simulink model "WMMSupportingForcesGP2021b"  (R2021b)
settings: Solver=ode23t  StartTime=0.0  StopTime=inf  FixedStep=.001  RelTol=1e-3  AbsTol=1e-3
InitFcn:
  | InitializeSimulationGP
  | SimulationParametersGP
values from neighbouring files (symbols this model uses):
  B11_r_B11C = [0.23805608; 0.13201777; 0]    [InitializeSimulationGP.m]
  B11_r_B11Tc1 = [L11; 0; 0]    [InitializeSimulationGP.m]
  B11_Rot_Tc1 = eye(3)    [InitializeSimulationGP.m]
  B11cI = [0.28426000 -0.06487287 0;         -0.06487287  0.54237481 0;                   0  0          0.67891020]    [InitializeSimulationGP.m]
  B12_r_B12C = [0.60504569; 0.27199376; 0.00002484]    [InitializeSimulationGP.m]
  B12_r_B12Tc2 = [L12;0;0]    [InitializeSimulationGP.m]
  B12_Rot_Tc2 = eye(3)    [InitializeSimulationGP.m]
  B12cI = [1.18803886 -2.36786418 0.00280315;          -2.36786418 6.31493281 0.00022322;           0.00280315 0.00022322 7.40915161]    [InitializeSimulationGP.m]
  B31_r_B31C = [0.35781210 0 0]    [InitializeSimulationGP.m]
  B31_Rot_B41 = eye(3)    [InitializeSimulationGP.m]
  B31cI = diag([0.03150902 0.90735702 0.90763033])    [InitializeSimulationGP.m]
  B32_r_B32C = [0.35781210 0 0]    [InitializeSimulationGP.m]
  B32_Rot_B42 = eye(3)    [InitializeSimulationGP.m]
  B32cI = diag([0.03150902 0.90735702 0.90763033])    [InitializeSimulationGP.m]
  B41_r_B41C = [0.55785997 0 0]    [InitializeSimulationGP.m]
  B41_r_B41Tc1 = [lc1;0;0]    [InitializeSimulationGP.m]
  B41cI = diag([0.00370720 0.55759812 0.55785997])    [InitializeSimulationGP.m]
  B42_r_B42C = [0.55785997 0 0]    [InitializeSimulationGP.m]
  B42_r_B42Tc2 = [lc2; 0; 0]    [InitializeSimulationGP.m]
  B42cI = diag([0.00370720 0.55759812 0.55785997])    [InitializeSimulationGP.m]
  B52_r_B52C = [0 0 0.56802906]    [InitializeSimulationGP.m]
  B52_r_B52P32 = [lc3; 0; 0]    [InitializeSimulationGP.m]
  B52_Rot_P32 = eye(3)    [InitializeSimulationGP.m]
  B52cI = diag([0.91789884, 0.91790043, 0.00091463])    [InitializeSimulationGP.m]
  Bc1_r_Bc1B11 = [L1; 0; 0]    [InitializeSimulationGP.m]
  Bc1_r_Bc1B31 = [0;0;0]    [InitializeSimulationGP.m]
  Bc1_r_Bc1C = [0.14178771; 0.16555780; 0]    [InitializeSimulationGP.m]
  Bc1_V = [0;0;0;0;0;0]    [InitializeSimulationGP.m]
  Bc1cI = [+5.892211080 +5.476111360 -0.000019630;          +5.476111360 +28.66965601 -0.000024550;          -0.000019630 -0.000024550 +29.78955950]    [InitializeSimulationGP.m]
  Bc2_r_Bc2B12 = [L2;0;0]    [InitializeSimulationGP.m]
  Bc2_r_Bc2B32 = [0;0;0]    [InitializeSimulationGP.m]
  Bc2_r_Bc2C = [0.54319901; 0.10543875; 0]    [InitializeSimulationGP.m]
  Bc2cI = [0.48071390 0.52924041 0;          0.52924041 5.80912352 0;              0      0          5.97255351]    [InitializeSimulationGP.m]
  BC_r_BCBM = [xCA; yCA; zCA]    [SimulationParametersGP.m]
  BC_Rot_BM = eye(3)    [SimulationParametersGP.m]
  BCI = diag([100 1200 1000])    [SimulationParametersGP.m]
  beta1 = atan2d(374.261,935)*pi/180    [InitializeSimulationGP.m]
  beta2 = atan2d(45.757,373.313)*pi/180    [InitializeSimulationGP.m]
  beta3 = atan2d(139.50,1132.19)*pi/180    [InitializeSimulationGP.m]
  beta4 = atan2d(88.061,296.198)*pi/180    [InitializeSimulationGP.m]
  betaGround = 1e6    (= 1000000)    [SimulationParametersGP.m]
  BFL = 0.05    [SimulationParametersGP.m]
  BFR = 0.05    [SimulationParametersGP.m]
  BM_r_BMBMp = [0;0;0]    [SimulationParametersGP.m]
  BM_Rot_BMp = [cos(gamma) -sin(gamma) 0; sin(gamma) cos(gamma) 0; 0 0 1]    [SimulationParametersGP.m]
  BMp_r_BMpBc1 = [0.185;0;0.205]    [InitializeSimulationGP.m]
  BMp_Rot_Bc1 = [cos(alpha1) -sin(alpha1)  0;                  0            0       -1;                sin(alpha1)  cos(alpha1)  0]    [InitializeSimulationGP.m]
  BRL = 0.05    [SimulationParametersGP.m]
  BRR = 0.05    [SimulationParametersGP.m]
  cc = 0.0    (= 0)    [SimulationParametersGP.m]
  D22F = [0;0;0;0;0;0]    [InitializeSimulationGP.m]
  dT = 0.01    [SimulationParametersGP.m]
  g0 = 9.8066    [SimulationParametersGP.m]
  ground_stiffness = 1e8    (= 100000000)    [SimulationParametersGP.m]
  l1 = 1.15-cc    (= 1.15)    [SimulationParametersGP.m]
  L1 = 1.0071227324212    (= 1.00712273242)    [InitializeSimulationGP.m]
  L11 = 0.37610632101293    (= 0.376106321013)    [InitializeSimulationGP.m]
  L12 = 0.30901132665325    (= 0.309011326653)    [InitializeSimulationGP.m]
  l2 = 1.15+cc    (= 1.15)    [SimulationParametersGP.m]
  L2 = 1.132185817991    (= 1.13218581799)    [InitializeSimulationGP.m]
  lc1 = 0.745    [InitializeSimulationGP.m]
  lc2 = 0.745    [InitializeSimulationGP.m]
  mB11 = 25.52660174    [InitializeSimulationGP.m]
  mB12 = 33.92850233    [InitializeSimulationGP.m]
  mB31 = 17.36281648    [InitializeSimulationGP.m]
  mB32 = 17.36281648    [InitializeSimulationGP.m]
  mB41 = 10.34519231    [InitializeSimulationGP.m]
  mB42 = 10.34519231    [InitializeSimulationGP.m]
  mB52 = 6.73059863    [InitializeSimulationGP.m]
  mBC = 2200    [SimulationParametersGP.m]
  mBc1 = 307.29601379    [InitializeSimulationGP.m]
  mBc2 = 54.58702836    [InitializeSimulationGP.m]
  mFL = 60    [SimulationParametersGP.m]
  mFR = 60    [SimulationParametersGP.m]
  mP22 = 9.26136143    [InitializeSimulationGP.m]
  mP32 = 570.18877059    [InitializeSimulationGP.m]
  mRR = 60    [SimulationParametersGP.m]
  mw = mFL    (= 60)    [SimulationParametersGP.m]
  P22_r_P22C = [0.62192523 0 0]    [InitializeSimulationGP.m]
  P22_Rot_B52 = eye(3)    [InitializeSimulationGP.m]
  P22cI = diag([0.00662754, 1.48387017, 1.48398069])    [InitializeSimulationGP.m]
  P32_r_P32C = [0.25466704; -0.13034397; -0.01302248]    [InitializeSimulationGP.m]
  P32_r_P32D22 = [0.40499744871392; -0.13130517281345; -0.013385243295654]    [InitializeSimulationGP.m]
  P32_Rot_D22 = [1 0 0;              0 0.9707729441837 0.23999977258512;              0 -0.23999977258512 0.9707729441837]    [InitializeSimulationGP.m]
  P32cI = [46.81220713 0.38607676 -0.00453819;          0.38607676 71.92201786 -1.14320993;          -0.00453819 -1.14320993 67.38128576]    [InitializeSimulationGP.m]
  R0FL = 0.35    [SimulationParametersGP.m]
  R0FR = 0.35    [SimulationParametersGP.m]
  R0RL = 0.35    [SimulationParametersGP.m]
  R0RR = 0.35    [SimulationParametersGP.m]
  Rw = R0FL    (= 0.35)    [SimulationParametersGP.m]
  Tc1_r_Tc1Bc2 = [0.098495302558553; 0.01838181329939; 0]    [InitializeSimulationGP.m]
  Tc1_Rot_Bc2 = [cos(alpha2) -sin(alpha2) 0;                sin(alpha2)  cos(alpha2) 0;                0            0           1]    [InitializeSimulationGP.m]
  Tc2_r_Tc2P22 = [-0.048858374920227;0.36587359346146;0.035276938723102]    [InitializeSimulationGP.m]
  Tc2_Rot_P22 = [0.95853460763586 -0.27664713597974  0.0683942111482;                0.28497614981675  0.93051946315663 -0.23004808784757;                0                 0.23999977258511  0.9707729441837]    [InitializeSimulationGP.m]
  Th1A = 10*pi/180    (= 0.174532925199)    [InitializeSimulationGP.m]
  Th1B = 20*pi/180    (= 0.349065850399)    [InitializeSimulationGP.m]
  Th1f = 1    [InitializeSimulationGP.m]
  Th2A = 15*pi/180    (= 0.261799387799)    [InitializeSimulationGP.m]
  Th2B = -70*pi/180    (= -1.2217304764)    [InitializeSimulationGP.m]
  Th2f = 2    [InitializeSimulationGP.m]
  w = wFL    (= 0.875)    [SimulationParametersGP.m]
  W_r_WBc1 = [0.185;0;0.205]    [InitializeSimulationGP.m]
  W_Rot_Bc1 = [cos(alpha1) -sin(alpha1)  0;                  0            0       -1;                sin(alpha1)  cos(alpha1)  0]    [InitializeSimulationGP.m]
  x10 = 0.83    [InitializeSimulationGP.m]
  x20 = 0.83    [InitializeSimulationGP.m]
  x3A = 0.2    [InitializeSimulationGP.m]
  x3B = 0.3    [InitializeSimulationGP.m]
  x3f = 1    [InitializeSimulationGP.m]
  xCA = 0.5    [SimulationParametersGP.m]
  xf = [1;0;0;0;0;0]    [InitializeSimulationGP.m]
  yCA = 0    [SimulationParametersGP.m]
  zC = 0.45    [SimulationParametersGP.m]
  zCA = .25    (= 0.25)    [SimulationParametersGP.m]
  ztau = [0;0;0;0;0;1]    [InitializeSimulationGP.m]
undefined symbols (not defined in the file or in its folder): alphaFL_meas, alphaFR_meas, alphaRL_meas, alphaRR_meas, B11_V, B11Ftot, B12_U_Tc2, B12_V, B12Ftot, B31_r_B31B41, B31_V, B31FTot, B32_r_B32B42, B32_U_B42, B32_V, B32FTot, B41_V, B41FTot, B42_Rot_Tc2, B42_U_Tc2, B42_V, B42FTot, B52_U_P32, B52_V, B52Ftot, Bc1Tot, Bc2_Rot_B12, Bc2_Rot_B32, Bc2_U_B12, Bc2_U_B32, Bc2_V, Bc2Tot, betaC_meas, D22_V, deltaFL_cmd, deltaFL_meas, deltaFR_cmd, deltaFR_meas, deltaRL_cmd, deltaRL_meas, deltaRR_cmd, deltaRR_meas, dOmegaFL_meas, dOmegaFR_meas, dOmegaRL_meas, dOmegaRR_meas, dPsi_meas, dq1, dq11, dq12, dq2, dq21, dq22, dx1, dx2, Floor, FTot_S1, FTot_S2P, FTot_S2R, FzFL ... (+63)
libraries: sm_lib x94, nesl_utility x63, simulink x5
(part 7 of 11)

== system WMMSupportingForcesGP2021b/Mobile Manipulator in Simscape/Hydraulic manipulator, Simscape/TiltCylinderAndTiltPiston ==
  B32Aux : sm_lib/Frames and Transforms/Rigid Transform  TranslationMethod=None  TranslationStandardOffset=0  TranslationLengthUnit=m  TranslationStandardAxis=+Z  TranslationCartesianOffset=[0 0 0]  TranslationROffset=0  TranslationROffsetUnits=m  TranslationZOffset=0  TranslationZOffsetUnits=m  TranslationThetaOffset=0  TranslationThetaOffsetUnits=deg  RotationMethod=StandardAxis  RotationAngleUnits=deg  RotationStandardAxis=+Y  RotationAngle=90  RotationArbitraryAxis=[0 0 1]  FollAlignAxisA=+X  BaseAlignAxisA=+Y  FollAlignAxisB=+Y  BaseAlignAxisB=+Z  RotationSequenceAxes=FollowerAxes  RotationSequence=XYX  RotationSequenceAngles=[0 0 0]  RotationSequenceAnglesUnits=deg  RotationMatrix=[1 0 0; 0 1 0; 0 0 1]
  B42Aux : sm_lib/Frames and Transforms/Rigid Transform  TranslationMethod=None  TranslationStandardOffset=0  TranslationLengthUnit=m  TranslationStandardAxis=+Z  TranslationCartesianOffset=[0 0 0]  TranslationROffset=0  TranslationROffsetUnits=m  TranslationZOffset=0  TranslationZOffsetUnits=m  TranslationThetaOffset=0  TranslationThetaOffsetUnits=deg  RotationMethod=StandardAxis  RotationAngleUnits=deg  RotationStandardAxis=+Y  RotationAngle=-90  RotationArbitraryAxis=[0 0 1]  FollAlignAxisA=+X  BaseAlignAxisA=+Y  FollAlignAxisB=+Y  BaseAlignAxisB=+Z  RotationSequenceAxes=FollowerAxes  RotationSequence=XYX  RotationSequenceAngles=[0 0 0]  RotationSequenceAnglesUnits=deg  RotationMatrix=[1 0 0; 0 1 0; 0 0 1]
  PS-Sim2 : nesl_utility/PS-Simulink Converter  PhysicalDomain=network_engine_domain  SubClassName=ps_output  LeftPortType=input  RightPortType=output  PseudoPeriodic=off  Frequencies=[]  Unit=inherit  AffineConversion=off
      settings: SourceProductBaseCode=PW,SS
  Tilt cylinder rotation (q21) : sm_lib/Joints/Revolute Joint  JointMode=Normal  SenseConstraintForce=off  SenseConstraintForceX=off  SenseConstraintForceY=off  SenseConstraintForceZ=off  SenseConstraintTorque=off  SenseConstraintTorqueX=off  SenseConstraintTorqueY=off  SenseConstraintTorqueZ=off  SenseTotalForce=off  SenseTotalForceX=off  SenseTotalForceY=off  SenseTotalForceZ=off  SenseTotalTorque=off  SenseTotalTorqueX=off  SenseTotalTorqueY=off  SenseTotalTorqueZ=off  CompositeWrenchDir=FollowerOnBase  CompositeWrenchFrame=BaseFrame  EquilibriumPosition=0  EquilibriumPositionUnits=deg  SpringStiffness=0  SpringStiffnessUnits=N*m/deg  DampingCoefficient=0  DampingCoefficientUnits=N*m/(deg/s)  TorqueActuationMode=NoTorque  MotionActuationMode=ComputedMotion  SensePosition=off  SenseVelocity=off  SenseAcceleration=off  SenseTorqueForce=off  SenseLowerLimitTorqueForce=off  SenseUpperLimitTorqueForce=off  LowerLimitSpecify=off  LowerLimitBound=-90  LowerLimitBoundUnits=deg  LowerLimitStiffness=1e4  LowerLimitStiffnessUnits=N*m/deg  LowerLimitDamping=10  LowerLimitDampingUnits=N*m/(deg/s)  LowerLimitTransitionRegionWidth=0.1  LowerLimitTransitionRegionWidthUnits=deg  UpperLimitSpecify=off  UpperLimitBound=90  UpperLimitBoundUnits=deg  UpperLimitStiffness=1e4  UpperLimitStiffnessUnits=N*m/deg  UpperLimitDamping=10  UpperLimitDampingUnits=N*m/(deg/s)  UpperLimitTransitionRegionWidth=0.1  UpperLimitTransitionRegionWidthUnits=deg  PositionTargetSpecify=off  PositionTargetPriority=High  PositionTargetValue=0  PositionTargetValueUnits=deg  VelocityTargetSpecify=off  VelocityTargetPriority=High  VelocityTargetValue=0  VelocityTargetValueUnits=deg/s
  Tilt piston rotation (q22) : sm_lib/Joints/Revolute Joint  JointMode=Normal  SenseConstraintForce=off  SenseConstraintForceX=off  SenseConstraintForceY=off  SenseConstraintForceZ=off  SenseConstraintTorque=off  SenseConstraintTorqueX=off  SenseConstraintTorqueY=off  SenseConstraintTorqueZ=off  SenseTotalForce=off  SenseTotalForceX=off  SenseTotalForceY=off  SenseTotalForceZ=off  SenseTotalTorque=off  SenseTotalTorqueX=off  SenseTotalTorqueY=off  SenseTotalTorqueZ=off  CompositeWrenchDir=FollowerOnBase  CompositeWrenchFrame=BaseFrame  EquilibriumPosition=0  EquilibriumPositionUnits=deg  SpringStiffness=0  SpringStiffnessUnits=N*m/deg  DampingCoefficient=0  DampingCoefficientUnits=N*m/(deg/s)  TorqueActuationMode=NoTorque  MotionActuationMode=ComputedMotion  SensePosition=off  SenseVelocity=off  SenseAcceleration=off  SenseTorqueForce=off  SenseLowerLimitTorqueForce=off  SenseUpperLimitTorqueForce=off  LowerLimitSpecify=off  LowerLimitBound=-90  LowerLimitBoundUnits=deg  LowerLimitStiffness=1e4  LowerLimitStiffnessUnits=N*m/deg  LowerLimitDamping=10  LowerLimitDampingUnits=N*m/(deg/s)  LowerLimitTransitionRegionWidth=0.1  LowerLimitTransitionRegionWidthUnits=deg  UpperLimitSpecify=off  UpperLimitBound=90  UpperLimitBoundUnits=deg  UpperLimitStiffness=1e4  UpperLimitStiffnessUnits=N*m/deg  UpperLimitDamping=10  UpperLimitDampingUnits=N*m/(deg/s)  UpperLimitTransitionRegionWidth=0.1  UpperLimitTransitionRegionWidthUnits=deg  PositionTargetSpecify=off  PositionTargetPriority=High  PositionTargetValue=0  PositionTargetValueUnits=deg  VelocityTargetSpecify=off  VelocityTargetPriority=High  VelocityTargetValue=0  VelocityTargetValueUnits=deg/s
  TiltCylinderSolid : sm_lib/Body Elements/File Solid  ExtGeomFileName=05_TiltCylGP.STEP  UnitType=FromFile  ExtGeomFileUnits=m  StepReaderType=OCC  ExportConvexHullGeometry=off  InertiaType=Custom  Mass=17.36281648  MassUnits=kg  CenterOfMass=[0 0.31781210 0]  CenterOfMassUnits=m  MomentsOfInertia=[0.90735702 0.03150902 0.90763033]  MomentsOfInertiaUnits=kg*m^2  ProductsOfInertia=[0 0 0]  ProductsOfInertiaUnits=kg*m^2  BasedOnType=Density  Density=7300  DensityUnits=kg/m^3  DoExposeReferenceFrame=off  SerializedFrames=<Frames><Frame><Id>Frame1</Id><Value><Name>B32</Name><Origin><Source>GeometricFeature</Source><FeatureName>cylindrical surface 11</FeatureName></Origin><PrimaryAxis><DefinedDirection>+X</DefinedDirection><Source>ReferenceFrame</Source><SourceDirection>+Y</SourceDirection><FeatureName></FeatureName></PrimaryAxis><SecondaryAxis><DefinedDirection>+Y</DefinedDirection><Source>ReferenceFrame</Source><SourceDirection>-X</SourceDirection><FeatureName></FeatureName></SecondaryAxis></Value></Frame><Frame><Id>Frame2</Id><Value><Name>B32Aux</Name><Origin><Source>GeometricFeature</Source><FeatureName>planar surface 4</FeatureName></Origin><PrimaryAxis><DefinedDirection>+X</DefinedDirection><Source>ReferenceFrame</Source><SourceDirection>+Y</SourceDirection><FeatureName></FeatureName></PrimaryAxis><SecondaryAxis><DefinedDirection>+Y</DefinedDirection><Source>ReferenceFrame</Source><SourceDirection>-X</SourceDirection><FeatureName></FeatureName></SecondaryAxis></Value></Frame></Frames>  GraphicType=FromGeometry  MarkerShape=Sphere  MarkerSize=10  GraphicVisPropType=SimpleVisualProperties  GraphicDiffuseColor=[1 1 119]/255  GraphicSpecularColor=[0.5 0.5 0.5 1.0]  GraphicAmbientColor=[0.15 0.15 0.15 1.0]  GraphicEmissiveColor=[0.0 0.0 0.0 1.0]  GraphicShininess=75  GraphicOpacity=1.0
  TiltPistonSolid : sm_lib/Body Elements/File Solid  ExtGeomFileName=06_TiltPistGP.STEP  UnitType=FromFile  ExtGeomFileUnits=m  StepReaderType=OCC  ExportConvexHullGeometry=off  InertiaType=Custom  Mass=10.34519231  MassUnits=kg  CenterOfMass=[0 0.32981882 0]  CenterOfMassUnits=m  MomentsOfInertia=[0.55759812 0.00370720 0.55785997]  MomentsOfInertiaUnits=kg*m^2  ProductsOfInertia=[0 0 0]  ProductsOfInertiaUnits=kg*m^2  BasedOnType=Density  Density=7850  DensityUnits=kg/m^3  DoExposeReferenceFrame=off  SerializedFrames=<Frames><Frame><Id>Frame2</Id><Value><Name>B42</Name><Origin><Source>GeometricFeature</Source><FeatureName>planar surface 2</FeatureName></Origin><PrimaryAxis><DefinedDirection>+X</DefinedDirection><Source>ReferenceFrame</Source><SourceDirection>+Y</SourceDirection><FeatureName></FeatureName></PrimaryAxis><SecondaryAxis><DefinedDirection>+Y</DefinedDirection><Source>ReferenceFrame</Source><SourceDirection>-X</SourceDirection><FeatureName></FeatureName></SecondaryAxis></Value></Frame><Frame><Id>Frame3</Id><Value><Name>P11</Name><Origin><Source>GeometricFeature</Source><FeatureName>cylindrical surface 8</FeatureName></Origin><PrimaryAxis><DefinedDirection>+X</DefinedDirection><Source>ReferenceFrame</Source><SourceDirection>+Y</SourceDirection><FeatureName></FeatureName></PrimaryAxis><SecondaryAxis><DefinedDirection>+Y</DefinedDirection><Source>ReferenceFrame</Source><SourceDirection>-X</SourceDirection><FeatureName></FeatureName></SecondaryAxis></Value></Frame></Frames>  GraphicType=FromGeometry  MarkerShape=Sphere  MarkerSize=10  GraphicVisPropType=SimpleVisualProperties  GraphicDiffuseColor=[9 232 232]/255  GraphicSpecularColor=[0.5 0.5 0.5 1.0]  GraphicAmbientColor=[0.15 0.15 0.15 1.0]  GraphicEmissiveColor=[0.0 0.0 0.0 1.0]  GraphicShininess=75  GraphicOpacity=1.0
  x2-translation : sm_lib/Joints/Prismatic Joint  JointMode=Normal  SenseConstraintForce=off  SenseConstraintForceX=off  SenseConstraintForceY=off  SenseConstraintForceZ=off  SenseConstraintTorque=off  SenseConstraintTorqueX=off  SenseConstraintTorqueY=off  SenseConstraintTorqueZ=off  SenseTotalForce=off  SenseTotalForceX=off  SenseTotalForceY=off  SenseTotalForceZ=off  SenseTotalTorque=off  SenseTotalTorqueX=off  SenseTotalTorqueY=off  SenseTotalTorqueZ=off  CompositeWrenchDir=FollowerOnBase  CompositeWrenchFrame=FollowerFrame  EquilibriumPosition=0  EquilibriumPositionUnits=m  SpringStiffness=0  SpringStiffnessUnits=N/m  DampingCoefficient=0  DampingCoefficientUnits=N/(m/s)  TorqueActuationMode=ComputedTorque  MotionActuationMode=ComputedMotion  SensePosition=off  SenseVelocity=off  SenseAcceleration=off  SenseTorqueForce=on  SenseLowerLimitTorqueForce=off  SenseUpperLimitTorqueForce=off  LowerLimitSpecify=off  LowerLimitBound=-1  LowerLimitBoundUnits=m  LowerLimitStiffness=1e6  LowerLimitStiffnessUnits=N/m  LowerLimitDamping=1e3  LowerLimitDampingUnits=N/(m/s)  LowerLimitTransitionRegionWidth=1e-4  LowerLimitTransitionRegionWidthUnits=m  UpperLimitSpecify=off  UpperLimitBound=1  UpperLimitBoundUnits=m  UpperLimitStiffness=1e6  UpperLimitStiffnessUnits=N/m  UpperLimitDamping=1e3  UpperLimitDampingUnits=N/(m/s)  UpperLimitTransitionRegionWidth=1e-4  UpperLimitTransitionRegionWidthUnits=m  PositionTargetSpecify=on  PositionTargetPriority=Low  PositionTargetValue=0.4  PositionTargetValueUnits=m  VelocityTargetSpecify=off  VelocityTargetPriority=High  VelocityTargetValue=0  VelocityTargetValueUnits=m/s
  B32 : PMIOPort  Side=Left
  B42 : PMIOPort  Port=2  Side=Left
  F4 : PMIOPort  Port=3  Side=Right
  F6 : PMIOPort  Port=4  Side=Right
  fc2 : Outport
  wires:
  PS-Sim2/1 -> fc2/1
  connections:
  TiltCylinderSolid/RConn1 -- B32Aux/LConn1
  x2-translation/RConn1 -- B42Aux/LConn1
  Tilt cylinder rotation (q21)/RConn1 -- TiltCylinderSolid/LConn1 -- B32/RConn1
  B42/RConn1 -- TiltPistonSolid/LConn1 -- B42Aux/RConn1
  B32Aux/RConn1 -- x2-translation/LConn1
  Tilt cylinder rotation (q21)/LConn1 -- F4/RConn1
  TiltPistonSolid/RConn1 -- Tilt piston rotation (q22)/LConn1
  Tilt piston rotation (q22)/RConn1 -- F6/RConn1
  PS-Sim2/LConn1 -- x2-translation/RConn2

== system WMMSupportingForcesGP2021b/Mobile Manipulator in Simscape/calc_betaC_from_meas/meas_VFL1 ==
  VFLx_meas : Inport
  VFLy_meas : Inport  Port=2
  Abs2 : Abs
  Atan : Trigonometry  Operator=atan
  Gain23 : Gain  Gain=1/BFL
  Integrator2 : Integrator
  Product3 : Product
  Sum9 : Sum  Inputs=|+-
  alphaFL_meas : Outport
  wires:
  Integrator2/1 -> Atan/1, Product3/1
  VFLy_meas/1 -> Sum9/1
  Sum9/1 -> Gain23/1
  Abs2/1 -> Product3/2
  VFLx_meas/1 -> Abs2/1
  Product3/1 -> Sum9/2
  Gain23/1 -> Integrator2/1
  Atan/1 -> alphaFL_meas/1

== system WMMSupportingForcesGP2021b/Mobile Manipulator in Simscape/meas_FLwheel_kinematic_quantities_in_Simscape/calc_longitudinal_slip_FL ==
  dOmegaFL_meas : Inport
  ReFL : Inport  Port=2
  VxFL_meas : Inport  Port=3
  Abs1 : Abs
  Gain : Gain  Gain=1e4
  Gain1 : Gain  Gain=1/BRL
  Integrator1 : Integrator
  Memory : Memory
  Product : Product  Inputs=3
  Product1 : Product  Inputs=3
  Product2 : Product
  Scope{,1..3} (4 alike) : Scope
  Sum1 : Sum  Inputs=|+-
  Sum2 : Sum  Inputs=|+-
  Tanh : Trigonometry  Operator=tanh
  kappaFL_meas : Outport
  wires:
  Product1/1 -> Scope2/1, Sum1/1
  Sum1/1 -> Scope1/1, Sum2/1
  Sum2/1 -> Gain1/1
  Product2/1 -> Sum2/2
  Gain1/1 -> Integrator1/1
  ReFL/1 -> Product1/2
  VxFL_meas/1 -> [VxFL_meas]
  [sgnVxFL] -> Product1/3
  [VxFL_meas] -> Abs1/1
  dOmegaFL_meas/1 -> Product1/1
  Abs1/1 -> Sum1/2, Scope3/1, Product2/2
  [sgnVxFL] -> Memory/1, Product/2
  Memory/1 -> Product/1
  Integrator1/1 -> Product/3
  Product/1 -> Product2/1, kappaFL_meas/1, Scope/1
  [VxFL_meas] -> Gain/1
  Gain/1 -> Tanh/1
  Tanh/1 -> [sgnVxFL]

== system WMMSupportingForcesGP2021b/Mobile Manipulator in Simscape/meas_FLwheel_kinematic_quantities_in_Simscape/meas_VFL ==
  VFLx_meas : Inport
  VFLy_meas : Inport  Port=2
  Product6 : Product
  Product7 : Product
  Sqrt : Sqrt  SaturateOnIntegerOverflow=on
  Sum16 : Sum  Inputs=|++
  VFL_meas : Outport
  wires:
  Product7/1 -> Sum16/2
  VFLx_meas/1 -> Product6/1, Product6/2
  Product6/1 -> Sum16/1
  VFLy_meas/1 -> Product7/1, Product7/2
  Sum16/1 -> Sqrt/1
  Sqrt/1 -> VFL_meas/1

== system WMMSupportingForcesGP2021b/Mobile Manipulator in Simscape/meas_FLwheel_kinematic_quantities_in_Simscape/meas_VFL1 ==
  VFLx_meas : Inport
  VFLy_meas : Inport  Port=2
  Abs2 : Abs
  Atan : Trigonometry  Operator=atan
  Gain23 : Gain  Gain=1/BFL
  Integrator2 : Integrator
  Product3 : Product
  Scope : Scope
  Sum9 : Sum  Inputs=|+-
  alphaFL_meas : Outport
  wires:
  Integrator2/1 -> Product3/1, Scope/1, Atan/1
  VFLy_meas/1 -> Sum9/1
  Sum9/1 -> Gain23/1
  Abs2/1 -> Product3/2
  VFLx_meas/1 -> Abs2/1
  Product3/1 -> Sum9/2
  Gain23/1 -> Integrator2/1
  Atan/1 -> alphaFL_meas/1

== system WMMSupportingForcesGP2021b/Mobile Manipulator in Simscape/meas_FRwheel_kinematic_quantities_in_Simscape/calc_longitudinal_slip_FR ==
  dOmegaFR_meas : Inport
  ReFR : Inport  Port=2
  VxFR_meas : Inport  Port=3
  Abs1 : Abs
  Gain : Gain  Gain=1e4
  Gain1 : Gain  Gain=1/BFR
  Integrator1 : Integrator
  Memory : Memory
  Product : Product  Inputs=3
  Product1 : Product  Inputs=3
  Product2 : Product
  Sum1 : Sum  Inputs=|+-
  Sum2 : Sum  Inputs=|+-
  Tanh : Trigonometry  Operator=tanh
  kappaFR_meas : Outport
  wires:
  Tanh/1 -> [sgnVxFR]
  [VxFR_meas] -> Gain/1
  VxFR_meas/1 -> [VxFR_meas]
  dOmegaFR_meas/1 -> Product1/1
  [sgnVxFR] -> Product1/3
  [VxFR_meas] -> Abs1/1
  Product2/1 -> Sum2/2
  Abs1/1 -> Sum1/2, Product2/2
  Gain1/1 -> Integrator1/1
  ReFR/1 -> Product1/2
  Sum1/1 -> Sum2/1
  Sum2/1 -> Gain1/1
  Product1/1 -> Sum1/1
  [sgnVxFR] -> Memory/1, Product/2
  Memory/1 -> Product/1
  Integrator1/1 -> Product/3
  Product/1 -> Product2/1, kappaFR_meas/1
  Gain/1 -> Tanh/1

== system WMMSupportingForcesGP2021b/Mobile Manipulator in Simscape/meas_FRwheel_kinematic_quantities_in_Simscape/meas_VFL1 ==
  VFRx_meas : Inport
  VFRy_meas : Inport  Port=2
  Abs2 : Abs
  Atan : Trigonometry  Operator=atan
  Gain23 : Gain  Gain=1/BFR
  Integrator2 : Integrator
  Product3 : Product
  Sum9 : Sum  Inputs=|+-
  alphaFR_meas : Outport
  wires:
  Integrator2/1 -> Atan/1, Product3/1
  Sum9/1 -> Gain23/1
  Abs2/1 -> Product3/2
  VFRx_meas/1 -> Abs2/1
  Product3/1 -> Sum9/2
  Gain23/1 -> Integrator2/1
  Atan/1 -> alphaFR_meas/1
  VFRy_meas/1 -> Sum9/1

== system WMMSupportingForcesGP2021b/Mobile Manipulator in Simscape/meas_FRwheel_kinematic_quantities_in_Simscape/meas_VFR ==
  VFRx_meas : Inport
  VFRy_meas : Inport  Port=2
  Product6 : Product
  Product7 : Product
  Sqrt : Sqrt  SaturateOnIntegerOverflow=on
  Sum16 : Sum  Inputs=|++
  VFR_meas : Outport
  wires:
  Sqrt/1 -> VFR_meas/1
  Sum16/1 -> Sqrt/1
  VFRy_meas/1 -> Product7/2, Product7/1
  Product6/1 -> Sum16/1
  VFRx_meas/1 -> Product6/2, Product6/1
  Product7/1 -> Sum16/2

== system WMMSupportingForcesGP2021b/Mobile Manipulator in Simscape/meas_RLwheel_kinematic_quantities_in_Simscape/calc_longitudinal_slip_RL ==
  dOmegaRL_meas : Inport
  ReRL : Inport  Port=2
  VxRL_meas : Inport  Port=3
  Abs1 : Abs
  Gain : Gain  Gain=1e4
  Gain1 : Gain  Gain=1/BRL
  Integrator1 : Integrator
  Memory : Memory
  Product : Product  Inputs=3
  Product1 : Product  Inputs=3
  Product2 : Product
  Sum1 : Sum  Inputs=|+-
  Sum2 : Sum  Inputs=|+-
  Tanh : Trigonometry  Operator=tanh
  kappaRL_meas : Outport
  wires:
  Product2/1 -> Sum2/2
  Sum2/1 -> Gain1/1
  Gain1/1 -> Integrator1/1
  ReRL/1 -> Product1/2
  Sum1/1 -> Sum2/1
  Abs1/1 -> Sum1/2, Product2/2
  dOmegaRL_meas/1 -> Product1/1
  Product1/1 -> Sum1/1
  [sgnVxRL] -> Product1/3
  VxRL_meas/1 -> [VxRL_meas]
  [VxRL_meas] -> Abs1/1
  Integrator1/1 -> Product/3
  [sgnVxRL] -> Memory/1, Product/2
  Memory/1 -> Product/1
  Product/1 -> Product2/1, kappaRL_meas/1
  [VxRL_meas] -> Gain/1
  Gain/1 -> Tanh/1
  Tanh/1 -> [sgnVxRL]

== system WMMSupportingForcesGP2021b/Mobile Manipulator in Simscape/meas_RLwheel_kinematic_quantities_in_Simscape/meas_VFL1 ==
  VRLx_meas : Inport
  VRLy_meas : Inport  Port=2
  Abs2 : Abs
  Atan : Trigonometry  Operator=atan
  Gain23 : Gain  Gain=1/BRL
  Integrator2 : Integrator
  Product3 : Product
  Scope : Scope
  Sum9 : Sum  Inputs=|+-
  alphaRL_meas : Outport
  wires:
  Integrator2/1 -> Atan/1, Product3/1
  VRLy_meas/1 -> Sum9/1
  Sum9/1 -> Gain23/1
  Abs2/1 -> Product3/2
  VRLx_meas/1 -> Abs2/1
  Product3/1 -> Sum9/2
  Gain23/1 -> Integrator2/1
  Atan/1 -> Scope/1, alphaRL_meas/1

== system WMMSupportingForcesGP2021b/Mobile Manipulator in Simscape/meas_RLwheel_kinematic_quantities_in_Simscape/meas_VRL ==
  VRLx_meas : Inport
  VRLy_meas : Inport  Port=2
  Product6 : Product
  Product7 : Product
  Sqrt : Sqrt  SaturateOnIntegerOverflow=on
  Sum16 : Sum  Inputs=|++
  VRL_meas : Outport
  wires:
  Sqrt/1 -> VRL_meas/1
  Sum16/1 -> Sqrt/1
  VRLy_meas/1 -> Product7/2, Product7/1
  Product6/1 -> Sum16/1
  VRLx_meas/1 -> Product6/2, Product6/1
  Product7/1 -> Sum16/2

== system WMMSupportingForcesGP2021b/Mobile Manipulator in Simscape/meas_RRwheel_kinematic_quantities_in_Simscape/calc_longitudinal_slip_RR ==
  dOmegaRR_meas : Inport
  ReRR : Inport  Port=2
  VxRR_meas : Inport  Port=3
  Abs1 : Abs
  Gain : Gain  Gain=1e4
  Gain1 : Gain  Gain=1/BRR
  Integrator1 : Integrator
  Memory : Memory
  Product : Product  Inputs=3
  Product1 : Product  Inputs=3
  Product2 : Product
  Sum1 : Sum  Inputs=|+-
  Sum2 : Sum  Inputs=|+-
  Tanh : Trigonometry  Operator=tanh
  kappaRR_meas : Outport
  wires:
  Product1/1 -> Sum1/1
  Sum1/1 -> Sum2/1
  Sum2/1 -> Gain1/1
  Product2/1 -> Sum2/2
  Gain1/1 -> Integrator1/1
  ReRR/1 -> Product1/2
  [sgnVxRR] -> Product1/3
  [VxRR_meas] -> Abs1/1
  dOmegaRR_meas/1 -> Product1/1
  Integrator1/1 -> Product/3
  Abs1/1 -> Sum1/2, Product2/2
  VxRR_meas/1 -> [VxRR_meas]
  Memory/1 -> Product/1
  [sgnVxRR] -> Memory/1, Product/2
  Product/1 -> kappaRR_meas/1, Product2/1
  [VxRR_meas] -> Gain/1
  Gain/1 -> Tanh/1
  Tanh/1 -> [sgnVxRR]

== system WMMSupportingForcesGP2021b/Mobile Manipulator in Simscape/meas_RRwheel_kinematic_quantities_in_Simscape/meas_VFL1 ==
  VRRx_meas : Inport
  VRRy_meas : Inport  Port=2
  Abs2 : Abs
  Atan : Trigonometry  Operator=atan
  Gain23 : Gain  Gain=1/BRR
  Integrator2 : Integrator
  Product3 : Product
  Sum9 : Sum  Inputs=|+-
  alphaRR_meas : Outport
  wires:
  Integrator2/1 -> Atan/1, Product3/1
  VRRy_meas/1 -> Sum9/1
  Sum9/1 -> Gain23/1
  Abs2/1 -> Product3/2
  Product3/1 -> Sum9/2
  Gain23/1 -> Integrator2/1
  Atan/1 -> alphaRR_meas/1
  VRRx_meas/1 -> Abs2/1

== system WMMSupportingForcesGP2021b/Mobile Manipulator in Simscape/meas_RRwheel_kinematic_quantities_in_Simscape/meas_VRR ==
  VRRx_meas : Inport
  VRRy_meas : Inport  Port=2
  Product6 : Product
  Product7 : Product
  Sqrt : Sqrt  SaturateOnIntegerOverflow=on
  Sum16 : Sum  Inputs=|++
  VRR_meas : Outport
  wires:
  Product7/1 -> Sum16/2
  VRRx_meas/1 -> Product6/1, Product6/2
  Product6/1 -> Sum16/1
  VRRy_meas/1 -> Product7/1, Product7/2
  Sum16/1 -> Sqrt/1
  Sqrt/1 -> VRR_meas/1

== system WMMSupportingForcesGP2021b/calc_wheel_velocities_and_sideslip_angles_from_meas/Hydraulic manipulator, calculation/AnalyticEnd-EffectorFramePosition ==
  note: Pass to outputs...
  note: Process data...
  note: Select from existing buses...
  note: Calculate end-effector position in the world frame...
  note: Get inputs...
  PosVecs_Sx : Inport
  WRotX_Sx : Inport  Port=2
  Bus Selector : BusSelector  OutputSignals=PosVecs_S1.W_r_WBc1,PosVecs_S1.Bc1_r_Bc1B11,PosVecs_S1.B11_r_B11Tc1,PosVecs_S1.Tc1_r_Tc1Bc2,PosVecs_S2R.Bc2_r_Bc2B12,PosVecs_S2R.B12_r_B12Tc2,PosVecs_S2R.Tc2_r_Tc2P22,PosVecs_S2P.P22_r_P22B52,PosVecs_S2P.B52_r_B52P32,PosVecs_S2P.P32_r_P32D22
  Bus Selector1 : BusSelector  OutputSignals=WRotX_S1.W_Rot_Bc1,WRotX_S1.W_Rot_B11,WRotX_S1.W_Rot_Tc1,WRotX_S1.W_Rot_Bc2,WRotX_S2R.W_Rot_B12,WRotX_S2R.W_Rot_Tc2,WRotX_S2R.W_Rot_P22,WRotX_S2P.W_Rot_B52,WRotX_S2P.W_Rot_P32
  Product{2..10} (9 alike) : Product  Multiplication=Matrix(*)
  Sum : Sum  Inputs=|++++++++++
  WrWD22 : Outport
  wires:
  WRotX_Sx/1 -> [WRotXSx]  "WRot_Sx"
  PosVecs_Sx/1 -> [PosVecsSx]  "PosVecs_Sx"
  [PosVecsSx] -> Bus Selector/1  "PosVecs_Sx"
  Bus Selector/2 -> [rBc1B11]  "<Bc1_r_Bc1B11>"
  Bus Selector/3 -> [rB11Tc1]  "<B11_r_B11Tc1>"
  Bus Selector/7 -> [rTc2P22]  "<Tc2_r_Tc2P22>"
  Bus Selector/6 -> [rB12Tc2]  "<B12_r_B12Tc2>"
  Bus Selector/5 -> [rBc2B12]  "<Bc2_r_Bc2B12>"
  Bus Selector/4 -> [rTc1Bc2]  "<Tc1_r_Tc1Bc2>"
  [rBc1B11] -> Product2/2
  [rB11Tc1] -> Product3/2
  [rTc1Bc2] -> Product4/2
  [rBc2B12] -> Product5/2
  [rB12Tc2] -> Product6/2
  [rTc2P22] -> Product7/2
  [WRotXSx] -> Bus Selector1/1  "WRotX_Sx"
  Bus Selector1/1 -> [WRotBc1]  "<W_Rot_Bc1>"
  Bus Selector1/2 -> [WRotB11]  "<W_Rot_B11>"
  Bus Selector1/3 -> [WRotTc1]  "<W_Rot_Tc1>"
  Bus Selector1/4 -> [WRotBc2]  "<W_Rot_Bc2>"
  Bus Selector1/5 -> [WRotB12]  "<W_Rot_B12>"
  Bus Selector1/6 -> [WRotTc2]  "<W_Rot_Tc2>"
  [WRotTc2] -> Product7/1
  [WRotB12] -> Product6/1
  [WRotBc2] -> Product5/1
  [WRotTc1] -> Product4/1
  [WRotB11] -> Product3/1
  [WRotBc1] -> Product2/1
  Sum/1 -> [WrWD22]  "WrWD22"
  [WrWD22] -> WrWD22/1  "WrWD22"
  Bus Selector1/7 -> [WRotP22]  "<W_Rot_P22>"
  Bus Selector1/8 -> [WRotB52]  "<W_Rot_B52>"
  Bus Selector/8 -> [rP22B52]  "<P22_r_P22B52>"
  Bus Selector/9 -> [rB52P32]  "<B52_r_B52P32>"
  [rP22B52] -> Product8/2
  [WRotP22] -> Product8/1
  [WRotB52] -> Product9/1
  [rB52P32] -> Product9/2
  Bus Selector1/9 -> [WRotP32]  "<W_Rot_P32>"
  Bus Selector/10 -> [rP32G]  "<P32_r_P32D22>"
  [rP32G] -> Product10/2
  [WRotP32] -> Product10/1
  Bus Selector/1 -> [rWBc1]  "<W_r_WBc1>"
  [rWBc1] -> Sum/1
  Product2/1 -> Sum/2
  Product3/1 -> Sum/3
  Product4/1 -> Sum/4
  Product5/1 -> Sum/5
  Product6/1 -> Sum/6
  Product7/1 -> Sum/7
  Product8/1 -> Sum/8
  Product9/1 -> Sum/9
  Product10/1 -> Sum/10

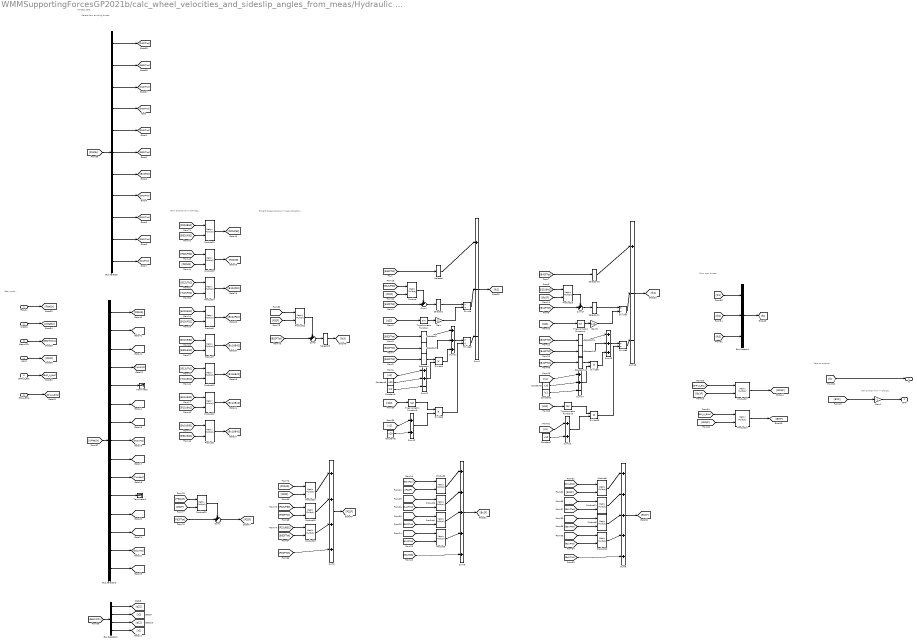
== system WMMSupportingForcesGP2021b/calc_wheel_velocities_and_sideslip_angles_from_meas/Hydraulic manipulator, calculation/AnalyticForces ==
  note: Manipulator Arm -> Chassis
  note: Pass to outputs...
  note: Form new buses...
  note: Process data...
  note: Extract forces acting on linear actuators...
  note: Form additional U matrices...
  note: Select from existing buses...
  note: Get inputs...
  Ftot_Sx : Inport
  UMatSx : Inport  Port=2
  GeomCCx : Inport  Port=3
  D22F : Inport  Port=4
  BMP_U_Bc1 : Inport  Port=5
  BM_U_BMp : Inport  Port=6
  Bus Creator1 : BusCreator  Inputs=3
  Bus Selector : BusSelector  OutputSignals=FTot_S2P.P32FTot,FTot_S2P.B52Ftot,FTot_S2P.P22FTot,FTot_S2R.B42FTot,FTot_S2R.B12Ftot,FTot_S2R.B32FTot,FTot_S2R.Bc2Tot,FTot_S1.B41FTot,FTot_S1.B11Ftot,FTot_S1.B31FTot,FTot_S1.Bc1Tot
  Bus Selector1 : BusSelector  OutputSignals=Geom_S2R.q22,Geom_S2R.x2,Geom_S1.q12,Geom_S1.x1
  Bus Selector2 : BusSelector  OutputSignals=UMats_S2P.P32_U_D22,UMats_S2P.B52_U_P32,UMats_S2P.P22_U_B52,UMats_S2R.Tc2_U_P22,UMats_S2R.B42_U_Tc2,UMats_S2R.B32_U_B42,UMats_S2R.Bc2_U_B32,UMats_S2R.B12_U_Tc2,UMats_S2R.Bc2_U_B12,UMats_S1.Tc1_U_Bc2,UMats_S1.B41_U_Tc1,UMats_S1.B31_U_B41,UMats_S1.Bc1_U_B31,UMats_S1.B11_U_Tc1,UMats_S1.Bc1_U_B11
  Constant1 : Constant  Value=lc2
  Constant2 : Constant  Value=lc1
  Constant3 : Constant  Value=x10
  Constant5 : Constant  Value=x20
  Constant6 : Constant  Value=x20
  Constant7 : Constant  Value=x10
  Divide{,5,7,9} (4 alike) : Product  Inputs=*/
  Divide{1,6,8,10} (4 alike) : Product  Inputs=**
  Gain : Gain  Gain=L12
  Gain1 : Gain  Gain=-1
  Gain5 : Gain  Gain=L11
  Product{,1..24} (25 alike) : Product  Multiplication=Matrix(*)
  Selector : Selector  InputPortWidth=6  IndexOptions=Index vector (dialog)  Indices=[1]  OutputSizes=1
  Selector{1..3,11..13} (6 alike) : Selector  InputPortWidth=6  IndexOptions=Index vector (dialog)  Indices=[6]  OutputSizes=1
  Selector10 : Selector  InputPortWidth=6  IndexOptions=Index vector (dialog)  Indices=[1]  OutputSizes=1
  Selector14 : Selector  InputPortWidth=6  IndexOptions=Index vector (dialog)  Indices=[2]  OutputSizes=1
  Selector4 : Selector  InputPortWidth=6  IndexOptions=Index vector (dialog)  Indices=[2]  OutputSizes=1
  Selector5 : Selector  InputPortWidth=6  IndexOptions=Index vector (dialog)  Indices=[1]  OutputSizes=1
  Sum1 : Sum  Inputs=|+--
  Sum10 : Sum  Inputs=|++-
  Sum11 : Sum  Inputs=|+++
  Sum12 : Sum  Inputs=|++
  Sum13 : Sum  Inputs=|+--
  Sum14 : Sum  Inputs=|++-
  Sum15 : Sum  Inputs=|+++
  Sum16 : Sum  Inputs=|++
  Sum{3..4,7,17} (4 alike) : Sum  Inputs=++|
  Sum2 : Sum  Inputs=|++++
  Sum5 : Sum  Inputs=|+++++
  Sum6 : Sum  Inputs=|+++++
  Terminator : Terminator
  Terminator1 : Terminator
  Trigonometric Function : Trigonometry
  Trigonometric Function3 : Trigonometry  Operator=tan
  Trigonometric Function4 : Trigonometry
  Trigonometric Function5 : Trigonometry  Operator=tan
  fc : Outport
  BMF : Outport  Port=2
  wires:
  Bus Selector/4 -> [B42FTot]  "<B42FTot>"
  Bus Selector/6 -> [B32FTot]  "<B32FTot>"
  Bus Selector/5 -> [B12FTot]  "<B12Ftot>"
  Bus Selector/7 -> [Bc2Tot]  "<Bc2Tot>"
  Bus Selector/8 -> [B41FTot]  "<B41FTot>"
  Bus Selector/9 -> [B11FTot]  "<B11Ftot>"
  Bus Selector/10 -> [B31FTot]  "<B31FTot>"
  Bus Selector/11 -> [Bc1FTot]  "<Bc1Tot>"
  [B42FTot] -> Selector/1
  Bus Selector1/1 -> [q22]  "<q22>"
  Bus Selector1/2 -> [x2]  "<x2>"
  Bus Selector1/4 -> [x1]  "<x1>"
  Bus Selector1/3 -> [q12]  "<q12>"
  Gain/1 -> Divide/2
  Trigonometric Function/1 -> Gain/1
  Selector/1 -> Sum1/1
  Divide/1 -> Sum1/2
  Sum1/1 -> [fc2]
  Bus Selector2/4 -> [Tc2UP22]  "<Tc2_U_P22>"
  Bus Selector2/5 -> Terminator/1  "<B42_U_Tc2>"
  Bus Selector2/6 -> [B32UB42]  "<B32_U_B42>"
  Bus Selector2/7 -> [Bc2UB32]  "<Bc2_U_B32>"
  Bus Selector2/8 -> [B12UTc2]  "<B12_U_Tc2>"
  Bus Selector2/9 -> [Bc2UB12]  "<Bc2_U_B12>"
  Bus Selector2/10 -> [Tc1UBc2]  "<Tc1_U_Bc2>"
  Bus Selector2/11 -> Terminator1/1  "<B41_U_Tc1>"
  Bus Selector2/12 -> [B31UB41]  "<B31_U_B41>"
  Bus Selector2/13 -> [Bc1UB31]  "<Bc1_U_B31>"
  Bus Selector2/14 -> [B11UTc1]  "<B11_U_Tc1>"
  Bus Selector2/15 -> [Bc1UB11]  "<Bc1_U_B11>"
  [B12FTot] -> Sum4/2
  Product/1 -> Sum4/1
  Sum4/1 -> Selector1/1
  [B12UP22] -> Product/1
  [Bc2UP22] -> Product3/1
  [P22F] -> Product/2
  [P22F] -> Product3/2
  Product3/1 -> Sum5/1
  [Bc2Tot] -> Sum5/5
  Product6/1 -> Sum5/2
  Product4/1 -> Sum5/3
  Product5/1 -> Sum5/4
  [B12FTot] -> Product5/2
  [Bc2UB12] -> Product5/1
  [B32FTot] -> Product4/2
  [B42FTot] -> Product6/2
  [B32UB42] -> Product7/2
  [Bc2UB32] -> Product7/1
  Product7/1 -> [Bc2UB42]
  [Bc2UB42] -> Product6/1
  [Bc2UB32] -> Product4/1
  Sum5/1 -> [Bc2F]
  Sum6/1 -> [Bc1F]
  [Bc1UB31] -> Product9/1
  [Bc1UB41] -> Product11/1
  [B41FTot] -> Product11/2
  [B31FTot] -> Product9/2
  [Bc1UB11] -> Product10/1
  [B11FTot] -> Product10/2
  Product10/1 -> Sum6/4
  Product9/1 -> Sum6/3
  Product11/1 -> Sum6/2
  [Bc1FTot] -> Sum6/5
  Product8/1 -> Sum6/1
  [Bc2F] -> Product8/2
  [Bc1UBc2] -> Product8/1
  Product1/1 -> [Bc2UP22]
  Product2/1 -> [Bc1UB41]
  [Bc1UB31] -> Product2/1
  [B31UB41] -> Product2/2
  [B12UTc2] -> Product14/1
  [Tc2UP22] -> Product14/2
  Product14/1 -> [B12UP22]
  [B12UP22] -> Product1/2
  [Bc2UB12] -> Product1/1
  [Bc1UB11] -> Product12/1
  [B11UBc2] -> Product12/2
  Product15/1 -> [B11UBc2]
  [Tc1UBc2] -> Product15/2
  [B11UTc1] -> Product15/1
  Product12/1 -> [Bc1UBc2]
  Selector1/1 -> Divide/1
  Divide5/1 -> Sum1/3
  Constant6/1 -> Sum12/2
  [x2] -> Sum12/1
  Selector2/1 -> Sum11/1
  Selector3/1 -> Sum11/2
  Divide1/1 -> Sum11/3
  [B32FTot] -> Selector2/1
  [B42FTot] -> Selector3/1
  [B42FTot] -> Selector4/1
  Selector4/1 -> Divide1/1
  Sum10/1 -> Divide1/2
  Constant1/1 -> Sum10/3
  [x2] -> Sum10/1
  Constant5/1 -> Sum10/2
  [fc1] -> Bus Creator1/1  "fc1"
  [fc2] -> Bus Creator1/2  "fc2"
  [q22] -> Trigonometric Function/1
  Ftot_Sx/1 -> [FtotSx]
  UMatSx/1 -> [UMatSx]
  GeomCCx/1 -> [GeomCCx]
  D22F/1 -> [D22F]
  [FtotSx] -> Bus Selector/1
  [UMatSx] -> Bus Selector2/1
  [GeomCCx] -> Bus Selector1/1
  Trigonometric Function3/1 -> Divide6/1
  Sum12/1 -> Divide6/2
  Sum11/1 -> Divide5/1
  Divide6/1 -> Divide5/2
  [q22] -> Trigonometric Function3/1
  [q12] -> Trigonometric Function5/1
  Divide10/1 -> Divide9/2
  Sum15/1 -> Divide9/1
  Sum16/1 -> Divide10/2
  Trigonometric Function5/1 -> Divide10/1
  [q12] -> Trigonometric Function4/1
  Constant3/1 -> Sum14/2
  [x1] -> Sum14/1
  Constant2/1 -> Sum14/3
  Sum14/1 -> Divide8/2
  Selector14/1 -> Divide8/1
  [B41FTot] -> Selector14/1
  [B41FTot] -> Selector13/1
  [B31FTot] -> Selector12/1
  Divide8/1 -> Sum15/3
  Selector13/1 -> Sum15/2
  Selector12/1 -> Sum15/1
  [x1] -> Sum16/1
  Constant7/1 -> Sum16/2
  Divide9/1 -> Sum13/3
  Selector11/1 -> Divide7/1
  [Bc2F] -> Product16/2
  [B11UBc2] -> Product16/1
  Sum17/1 -> Selector11/1
  Product16/1 -> Sum17/1
  [B11FTot] -> Sum17/2
  Sum13/1 -> [fc1]
  Divide7/1 -> Sum13/2
  Selector10/1 -> Sum13/1
  Trigonometric Function4/1 -> Gain5/1
  Gain5/1 -> Divide7/2
  [B41FTot] -> Selector10/1
  Bus Creator1/1 -> [fc]
  [fc] -> fc/1
  Bus Selector/3 -> [P22FTot]  "<P22FTot>"
  Bus Selector/2 -> [B52FTot]  "<B52Ftot>"
  Bus Selector/1 -> [P32FTot]  "<P32FTot>"
  Bus Selector2/1 -> [P32UG]  "<P32_U_D22>"
  Bus Selector2/3 -> [P22UB52]  "<P22_U_B52>"
  Bus Selector2/2 -> [B52UP32]  "<B52_U_P32>"
  Sum2/1 -> [P22F]
  Product18/1 -> Sum2/2
  [P22FTot] -> Sum2/4
  Product19/1 -> Sum2/3
  Product20/1 -> Sum2/1
  [B52FTot] -> Product19/2
  [P32FTot] -> Product18/2
  [D22F] -> Product20/2
  [P22UG] -> Product20/1
  [P22UB52] -> Product21/1
  [B52UP32] -> Product21/2
  Product21/1 -> [P22UP32]
  [P22UP32] -> Product18/1
  [P22UB52] -> Product19/1
  [B52FTot] -> Sum3/2
  Product22/1 -> Sum3/1
  [P32FTot] -> Sum7/2
  [D22F] -> Product23/2
  [P32UG] -> Product23/1
  Product23/1 -> Sum7/1
  Sum7/1 -> [P32F]
  [P32F] -> Product22/2
  [B52UP32] -> Product22/1
  Sum3/1 -> Selector5/1
  Selector5/1 -> [fc3]
  [fc3] -> Bus Creator1/3  "fc3"
  [Bc1F] -> Product17/2  "Bc1F"
  Product13/1 -> [P22UG]
  [P32UG] -> Product13/2
  [P22UP32] -> Product13/1
  [BMP_U_Bc1] -> Product17/1  "BMp_U_Bc1"
  Product17/1 -> [BMpF]  "BMpF"
  [BM_U_BMp] -> Product24/1  "BM_U_BMp"
  [BMpF] -> Product24/2  "BMpF"
  Product24/1 -> [BMF]  "BMF"
  BMP_U_Bc1/1 -> [BMP_U_Bc1]
  BM_U_BMp/1 -> [BM_U_BMp]
  [BMF] -> Gain1/1
  Gain1/1 -> BMF/1

== system WMMSupportingForcesGP2021b/calc_wheel_velocities_and_sideslip_angles_from_meas/Hydraulic manipulator, calculation/AnalyticTotalForces ==
  note: Process data...
  note: Pass to outputs...
  note: Get inputs...
  Vels_Sx : Inport
  WRotX_Sx : Inport  Port=2
  Bus Creator : BusCreator  Inputs=FTot_S1,FTot_S2R,FTot_S2P
  Structure 1 : Subsystem
  Structure 2 (Prismatic segment) : Subsystem
  Structure 2 (Revolute segment) : Subsystem
  FTot_Sx : Outport
  wires:
  Vels_Sx/1 -> [VelsSx]
  WRotX_Sx/1 -> [WRotSx]
  [VelsSx] -> Structure 1/1(Vels_Sx)
  [VelsSx] -> Structure 2 (Revolute segment)/1(Vels_Sx)
  [WRotSx] -> Structure 1/2(WRotX_Sx)
  [WRotSx] -> Structure 2 (Revolute segment)/2(WRotX_Sx)
  Structure 2 (Revolute segment)/1(FTot_S2R) -> [FTotS2R]
  Structure 1/1(FTot_S1) -> [FTotS1]
  [FTotS2R] -> Bus Creator/2  "FTot_S2R"
  [FTotS1] -> Bus Creator/1  "FTot_S1"
  [FTotSx] -> FTot_Sx/1  "FTot_Sx"
  Bus Creator/1 -> [FTotSx]
  [WRotSx] -> Structure 2 (Prismatic segment)/2(WRotX_Sx)
  [VelsSx] -> Structure 2 (Prismatic segment)/1(Vels_Sx)
  Structure 2 (Prismatic segment)/1(FTot_S2P) -> [FTotS2P]
  [FTotS2P] -> Bus Creator/3  "FTot_S2P"

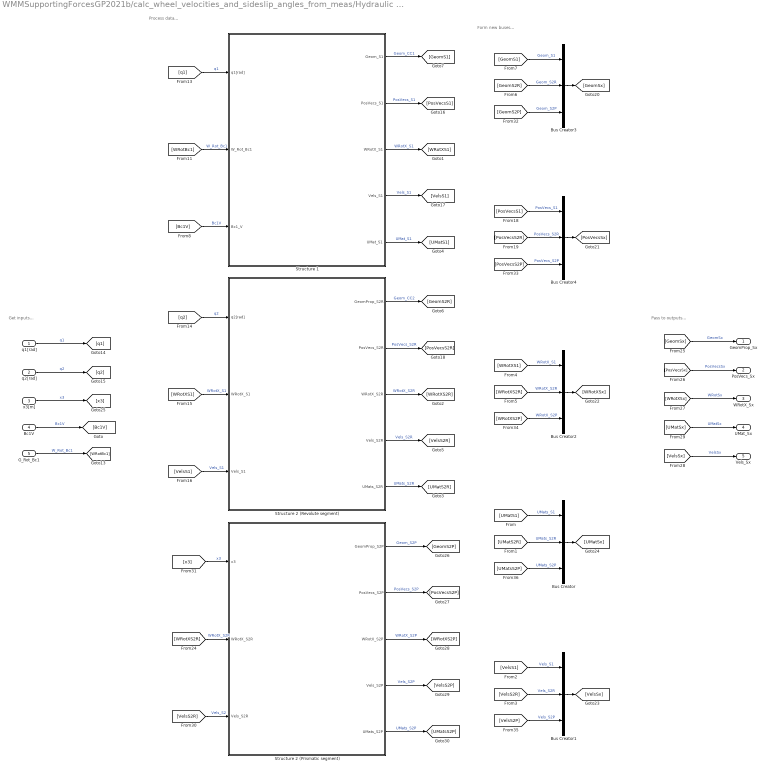
== system WMMSupportingForcesGP2021b/calc_wheel_velocities_and_sideslip_angles_from_meas/Hydraulic manipulator, calculation/AnalyticVelocities ==
  note: Pass to outputs...
  note: Form new buses...
  note: Process data...
  note: Get inputs...
  q1[rad] : Inport  Unit=rad
  q2[rad] : Inport  Port=2
  x3[m] : Inport  Port=3
  Bc1V : Inport  Port=4
  G_Rot_Bc1 : Inport  Port=5
  Bus Creator{,1..4} (5 alike) : BusCreator  Inputs=3
  Structure 1 : Subsystem
  Structure 2 (Prismatic segment) : Subsystem
  Structure 2 (Revolute segment) : Subsystem
  GeomProp_Sx : Outport
  PosVecs_Sx : Outport  Port=2
  WRotX_Sx : Outport  Port=3
  UMat_Sx : Outport  Port=4
  Vels_Sx : Outport  Port=5
  wires:
  Structure 1/4(Vels_S1) -> [VelsS1]  "Vels_S1"
  [VelsS1] -> Structure 2 (Revolute segment)/3(Vels_S1)  "Vels_S1"
  Structure 2 (Revolute segment)/4(Vels_S2R) -> [VelsS2R]  "Vels_S2R"
  Structure 2 (Revolute segment)/5(UMats_S2R) -> [UMatS2R]  "UMats_S2R"
  Structure 1/5(UMat_S1) -> [UMatS1]  "UMat_S1"
  Structure 1/3(WRotX_S1) -> [WRotXS1]  "WRotX_S1"
  [WRotXS1] -> Structure 2 (Revolute segment)/2(WRotX_S1)  "WRotX_S1"
  Structure 2 (Revolute segment)/3(WRotX_S2R) -> [WRotXS2R]  "WRotX_S2R"
  Structure 2 (Revolute segment)/1(GeomProp_S2R) -> [GeomS2R]  "Geom_CC2"
  Structure 1/1(Geom_S1) -> [GeomS1]  "Geom_CC1"
  G_Rot_Bc1/1 -> [WRotBc1]  "W_Rot_Bc1"
  [WRotBc1] -> Structure 1/2(W_Rot_Bc1)  "W_Rot_Bc1"
  [Bc1V] -> Structure 1/3(Bc1_V)  "Bc1V"
  q1[rad]/1 -> [q1]  "q1"
  [q1] -> Structure 1/1(q1[rad])  "q1"
  q2[rad]/1 -> [q2]  "q2"
  [q2] -> Structure 2 (Revolute segment)/1(q2[rad])  "q2"
  Structure 1/2(PosVecs_S1) -> [PosVecsS1]  "PosVecs_S1"
  [PosVecsS1] -> Bus Creator4/1  "PosVecs_S1"
  Structure 2 (Revolute segment)/2(PosVecs_S2R) -> [PosVecsS2R]  "PosVecs_S2R"
  [PosVecsS2R] -> Bus Creator4/2  "PosVecs_S2R"
  [WRotXS2R] -> Bus Creator2/2  "WRotX_S2R"
  [WRotXS1] -> Bus Creator2/1  "WRotX_S1"
  [UMatS2R] -> Bus Creator/2  "UMats_S2R"
  [UMatS1] -> Bus Creator/1  "UMats_S1"
  [VelsS1] -> Bus Creator1/1  "Vels_S1"
  [VelsS2R] -> Bus Creator1/2  "Vels_S2R"
  [GeomS2R] -> Bus Creator3/2  "Geom_S2R"
  [GeomS1] -> Bus Creator3/1  "Geom_S1"
  Bus Creator3/1 -> [GeomSx]
  Bus Creator4/1 -> [PosVecsSx]
  Bus Creator2/1 -> [WRotXSx]
  Bus Creator1/1 -> [VelsSx]
  Bus Creator/1 -> [UMatSx]
  [GeomSx] -> GeomProp_Sx/1  "GeomSx"
  [PosVecsSx] -> PosVecs_Sx/1  "PosVecsSx"
  [WRotXSx] -> WRotX_Sx/1  "WRotSx"
  [VelsSx] -> Vels_Sx/1  "VelsSx"
  [UMatSx] -> UMat_Sx/1  "UMatSx"
  x3[m]/1 -> [x3]  "x3"
  [x3] -> Structure 2 (Prismatic segment)/1(x3)  "x3"
  [WRotXS2R] -> Structure 2 (Prismatic segment)/2(WRotX_S2R)  "WRotX_S2R"
  [VelsS2R] -> Structure 2 (Prismatic segment)/3(Vels_S2R)  "Vels_S2"
  Structure 2 (Prismatic segment)/1(GeomProp_S2P) -> [GeomS2P]  "Geom_S2P"
  [GeomS2P] -> Bus Creator3/3  "Geom_S2P"
  Structure 2 (Prismatic segment)/2(PosVecs_S2P) -> [PosVecsS2P]  "PosVecs_S2P"
  [PosVecsS2P] -> Bus Creator4/3  "PosVecs_S2P"
  Structure 2 (Prismatic segment)/3(WRotX_S2P) -> [WRotXS2P]  "WRotX_S2P"
  [WRotXS2P] -> Bus Creator2/3  "WRotX_S2P"
  Structure 2 (Prismatic segment)/4(Vels_S2P) -> [VelsS2P]  "Vels_S2P"
  Structure 2 (Prismatic segment)/5(UMats_S2P) -> [UMatsS2P]  "UMats_S2P"
  [UMatsS2P] -> Bus Creator/3  "UMats_S2P"
  [VelsS2P] -> Bus Creator1/3  "Vels_S2P"
  Bc1V/1 -> [Bc1V]  "Bc1V"

== system WMMSupportingForcesGP2021b/calc_wheel_velocities_and_sideslip_angles_from_meas/Hydraulic manipulator, calculation/AngleRelations ==
  note: Pass to outputs...
  note: Process data...
  note: Get inputs...
  note: Calculate q1 and q2 from Theta1 and Theta2...
  Theta1[rad] : Inport
  Theta2[rad] : Inport  Port=2
  Fcn : Fcn  Expr=-pi/2 - beta1 - beta2 + u
  Fcn1 : Fcn  Expr=+u - beta3 - beta4
  q1[rad] : Outport
  q2[rad] : Outport  Port=2
  wires:
  Theta1[rad]/1 -> [Theta1]
  Theta2[rad]/1 -> [Theta2]
  [Theta2] -> Fcn1/1
  [Theta1] -> Fcn/1
  Fcn/1 -> [q1]
  [q1] -> q1[rad]/1
  [q2] -> q2[rad]/1
  Fcn1/1 -> [q2]

== system WMMSupportingForcesGP2021b/Mobile Manipulator in Simscape/GroundReactionFL/verticalForceFL/dampingForceFL ==
  note: Apply damping only when stiffness force >0
  Fz k : Inport
  vz : Inport  Port=2
  Constant : Constant  Value=0
  Constant1 : Constant  Value=betaGround
  Product : Product
  Saturation : Saturate  UpperLimit=0  LowerLimit=-Inf
  Switch : Switch  Criteria=u2 > Threshold  ZeroCross=off
  Fz d : Outport  VectorParamsAs1DForOutWhenUnconnected=off
  wires:
  Product/1 -> Switch/1
  Fz k/1 -> Switch/2
  Switch/1 -> Fz d/1
  Constant/1 -> Switch/3
  Constant1/1 -> Product/2
  vz/1 -> Saturation/1
  Saturation/1 -> Product/1

== system WMMSupportingForcesGP2021b/Mobile Manipulator in Simscape/GroundReactionFR/verticalForceFR/dampingForceFR ==
  note: Apply damping only when stiffness force >0
  Fz k : Inport
  vz : Inport  Port=2
  Constant : Constant  Value=0
  Constant1 : Constant  Value=betaGround
  Product : Product
  Saturation : Saturate  UpperLimit=0  LowerLimit=-Inf
  Switch : Switch  Criteria=u2 > Threshold  ZeroCross=off
  Fz d : Outport  VectorParamsAs1DForOutWhenUnconnected=off
  wires:
  Product/1 -> Switch/1
  Fz k/1 -> Switch/2
  Switch/1 -> Fz d/1
  Constant/1 -> Switch/3
  Constant1/1 -> Product/2
  vz/1 -> Saturation/1
  Saturation/1 -> Product/1

== system WMMSupportingForcesGP2021b/Mobile Manipulator in Simscape/GroundReactionRL/verticalForceRL/dampingForceRL ==
  note: Apply damping only when stiffness force >0
  Fz k : Inport
  vz : Inport  Port=2
  Constant : Constant  Value=0
  Constant1 : Constant  Value=betaGround
  Product : Product
  Saturation : Saturate  UpperLimit=0  LowerLimit=-Inf
  Switch : Switch  Criteria=u2 > Threshold  ZeroCross=off
  Fz d : Outport  VectorParamsAs1DForOutWhenUnconnected=off
  wires:
  Product/1 -> Switch/1
  Fz k/1 -> Switch/2
  Switch/1 -> Fz d/1
  Constant/1 -> Switch/3
  Constant1/1 -> Product/2
  vz/1 -> Saturation/1
  Saturation/1 -> Product/1

== system WMMSupportingForcesGP2021b/Mobile Manipulator in Simscape/GroundReactionRR/verticalForceRR/dampingForceRR ==
  note: Apply damping only when stiffness force >0
  Fz k : Inport
  vz : Inport  Port=2
  Constant : Constant  Value=0
  Constant1 : Constant  Value=betaGround
  Product : Product
  Saturation : Saturate  UpperLimit=0  LowerLimit=-Inf
  Switch : Switch  Criteria=u2 > Threshold  ZeroCross=off
  Fz d : Outport  VectorParamsAs1DForOutWhenUnconnected=off
  wires:
  Product/1 -> Switch/1
  Fz k/1 -> Switch/2
  Switch/1 -> Fz d/1
  Constant/1 -> Switch/3
  Constant1/1 -> Product/2
  vz/1 -> Saturation/1
  Saturation/1 -> Product/1
